simulink model "TwoToFourDecoder"  (R2017b)
settings: Solver=VariableStepAuto  StartTime=0.0  StopTime=10.0  RelTol=1e-3
settings Model: Creator=Ray  LastModifiedBy=Ray

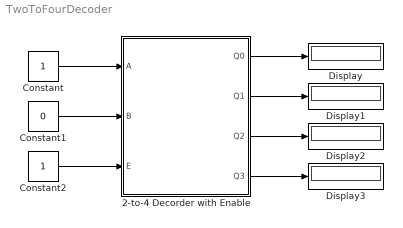
== system TwoToFourDecoder ==
  2-to-4 Decorder with Enable : Subsystem
  Constant : Constant  OutDataTypeStr=boolean  SampleTime=1
  Constant1 : Constant  Value=0  OutDataTypeStr=boolean  SampleTime=1
  Constant2 : Constant  OutDataTypeStr=boolean  SampleTime=1
  Display{,1..3} (4 alike) : Display
  wires:
  Constant/1 -> 2-to-4 Decorder with Enable/1(A)
  Constant1/1 -> 2-to-4 Decorder with Enable/2(B)
  Constant2/1 -> 2-to-4 Decorder with Enable/3(E)
  2-to-4 Decorder with Enable/1(Q0) -> Display/1
  2-to-4 Decorder with Enable/2(Q1) -> Display1/1
  2-to-4 Decorder with Enable/3(Q2) -> Display2/1
  2-to-4 Decorder with Enable/4(Q3) -> Display3/1

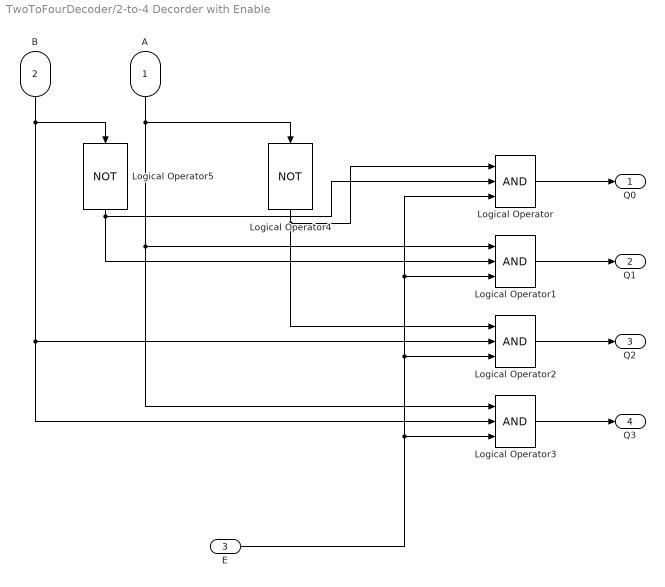
== system TwoToFourDecoder/2-to-4 Decorder with Enable ==
  A : Inport  OutDataTypeStr=boolean  SampleTime=1
  B : Inport  Port=2  OutDataTypeStr=boolean  SampleTime=1
  E : Inport  Port=3  OutDataTypeStr=boolean  SampleTime=1
  Logical Operator{,1..3} (4 alike) : Logic  Inputs=3  IconShape=distinctive  AllPortsSameDT=off  OutDataTypeStr=boolean
  Logical Operator4 : Logic  Operator=NOT  Inputs=3  IconShape=distinctive  AllPortsSameDT=off  OutDataTypeStr=boolean
  Logical Operator5 : Logic  Operator=NOT  Inputs=3  IconShape=distinctive  AllPortsSameDT=off  OutDataTypeStr=boolean
  Q0 : Outport  SampleTime=1
  Q1 : Outport  Port=2  SampleTime=1
  Q2 : Outport  Port=3  SampleTime=1
  Q3 : Outport  Port=4  SampleTime=1
  wires:
  Logical Operator5/1 -> Logical Operator1/2, Logical Operator/2
  Logical Operator2/1 -> Q2/1
  Logical Operator4/1 -> Logical Operator2/1, Logical Operator/1
  Logical Operator3/1 -> Q3/1
  Logical Operator1/1 -> Q1/1
  Logical Operator/1 -> Q0/1
  A/1 -> Logical Operator1/1, Logical Operator3/1, Logical Operator4/1
  B/1 -> Logical Operator2/2, Logical Operator3/2, Logical Operator5/1
  E/1 -> Logical Operator3/3, Logical Operator2/3, Logical Operator1/3, Logical Operator/3
